simulink model "tp1"  (R2017b)
settings: Solver=VariableStepAuto  StartTime=0.0  StopTime=10.0  RelTol=1e-3
values from neighbouring files (symbols this model uses):
  A = [0 1 0;0 0 1;-2 -5 -4]    [TP1.m]
  a1 = 10    [TP1.m]
  a2 = 20    [TP1.m]
  a3 = 40    [TP1.m]
  B = [0;0;1]    [TP1.m]
  C = [1 0 0]    [TP1.m]
  F = exp(1)^A*T    [TP1.m]
  H = C    [TP1.m]
  L = [place(A',C',P)]'    [TP1.m]
  l1 = 25    [TP1.m]
  l2 = 20    [TP1.m]
  l3 = 35    [TP1.m]
undefined symbols (not defined in the file or in its folder): G
libraries: dspsrcs4 x2
settings Model: Creator=dell 15  LastModifiedBy=bo199

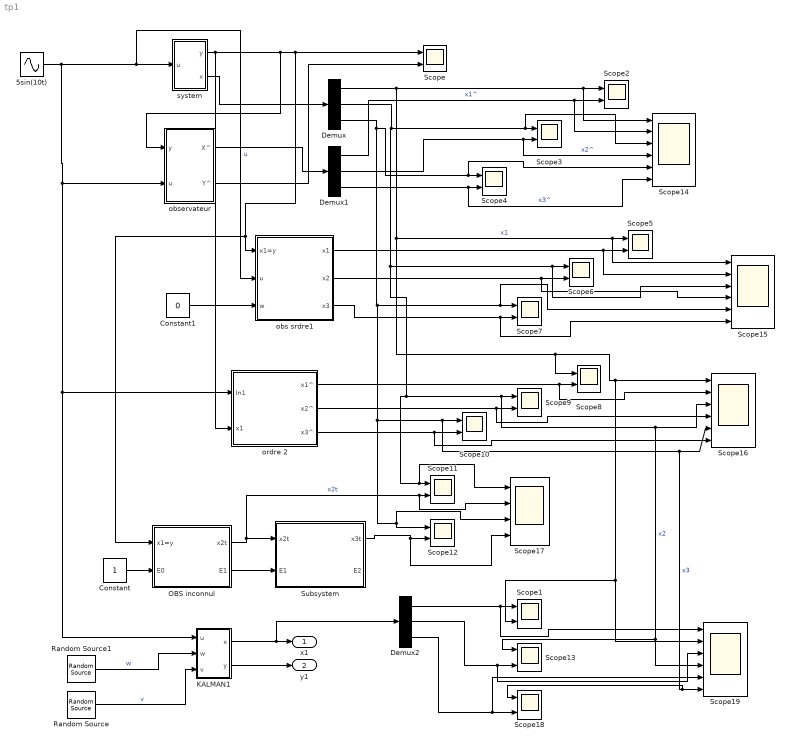
== system tp1 ==
  5sin(10t) : Sin  Amplitude=5  Frequency=10  SampleTime=0
  Constant : Constant
  Constant1 : Constant  Value=0
  Demux : Demux  Outputs=3
  Demux1 : Demux  Outputs=3
  Demux2 : Demux  Outputs=3
  KALMAN1 : Subsystem
  OBS inconnul : Subsystem
  Random Source : dspsrcs4/Random Source  SrcType=Uniform  NormMethod=Ziggurat  CltLength=12  MinVal=0  MaxVal=1  MeanVal=0  VarVal=1  RepMode=Not repeatable  rawSeed=1  IsInherit=off  SampMode=Discrete  SampTime=1  SampFrame=1  DataType=Double  OutComplex=Real  OutputFrames=off
  Random Source1 : dspsrcs4/Random Source  SrcType=Uniform  NormMethod=Ziggurat  CltLength=12  MinVal=0  MaxVal=1  MeanVal=0  VarVal=1  RepMode=Not repeatable  rawSeed=1  IsInherit=off  SampMode=Discrete  SampTime=1  SampFrame=1  DataType=Double  OutComplex=Real  OutputFrames=off
  Scope{,1..13,18} (15 alike) : Scope  NumInputPorts=2
  Scope{14..16,19} (4 alike) : Scope  NumInputPorts=6
  Scope17 : Scope  NumInputPorts=4
  Subsystem : Subsystem
  obs srdre1 : Subsystem
  observateur : Subsystem
  "ordre 2 " : Subsystem
  system : Subsystem
  x1 : Outport
  y1 : Outport  Port=2
  wires:
  system/1(y) -> Scope/1, OBS inconnul/1(x1=y), obs srdre1/1(x1=y), observateur/1(y), "ordre 2 "/2("x1 ")
  5sin(10t)/1 -> "ordre 2 "/1(In1), KALMAN1/1(u), observateur/2(u), obs srdre1/2(u), system/1("u ")  "u"
  system/2(x) -> Demux/1
  observateur/2(Y^) -> Scope/2
  OBS inconnul/1(x2t) -> Subsystem/1(x2t), Scope17/2, Scope11/2  "x2t"
  OBS inconnul/2(E1) -> Subsystem/2(E1)
  Constant/1 -> OBS inconnul/2(E0)
  Random Source1/1 -> KALMAN1/2(w)  "w"
  Random Source/1 -> KALMAN1/3(v)  "v"
  KALMAN1/2(y) -> y1/1
  Demux/3 -> Scope17/3, Scope12/1, Scope18/1, Scope19/6, Scope16/5, Scope10/1, Scope15/5, Scope7/1, Scope14/5, Scope4/1  "x3"
  Demux/2 -> Scope19/4, Scope13/1, Scope16/3, Scope9/1, Scope17/1, Scope11/1, Scope15/3, Scope6/1, Scope14/3, Scope3/1  "x2"
  Demux/1 -> Scope8/1, Scope19/2, Scope1/2, Scope16/1, Scope15/1, Scope5/1, Scope14/1, Scope2/1  "x1"
  observateur/1(X^) -> Demux1/1
  Demux1/1 -> Scope14/2, Scope2/2  "x1^"
  Demux1/2 -> Scope14/4, Scope3/2  "x2^"
  Demux1/3 -> Scope14/6, Scope4/2  "x3^"
  obs srdre1/1(x1) -> Scope15/2, Scope5/2
  obs srdre1/2(x2) -> Scope15/4, Scope6/2
  obs srdre1/3(x3) -> Scope15/6, Scope7/2
  "ordre 2 "/1(x1^) -> Scope16/2, Scope8/2
  "ordre 2 "/2(x2^) -> Scope16/4, Scope9/2
  "ordre 2 "/3(x3^) -> Scope16/6, Scope10/2
  Constant1/1 -> obs srdre1/3(w)
  Subsystem/1(x3t) -> Scope17/4, Scope12/2
  KALMAN1/1(x) -> Demux2/1, x1/1
  Demux2/1 -> Scope19/1, Scope1/1
  Demux2/2 -> Scope19/3, Scope13/2
  Demux2/3 -> Scope19/5, Scope18/2

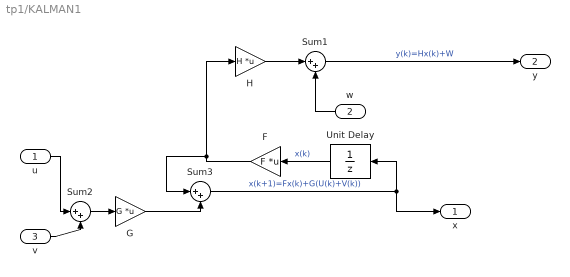
== system tp1/KALMAN1 ==
  u : Inport
  w : Inport  Port=2
  v : Inport  Port=3
  F : Gain  Gain=F  Multiplication=Matrix(K*u)
  G : Gain  Gain=G  Multiplication=Matrix(K*u)
  H : Gain  Gain=H  Multiplication=Matrix(K*u)
  Sum1 : Sum  Inputs=|++
  Sum2 : Sum  Inputs=|++
  Sum3 : Sum  Inputs=|++
  Unit Delay : UnitDelay  SampleTime=-1
  x : Outport
  y : Outport  Port=2
  wires:
  Sum3/1 -> x/1, Unit Delay/1  "x(k+1)=Fx(k)+G(U(k)+V(k))"
  F/1 -> H/1, Sum3/1
  u/1 -> Sum2/1
  Sum1/1 -> y/1  "y(k)=Hx(k)+W"
  H/1 -> Sum1/1
  G/1 -> Sum3/2
  Unit Delay/1 -> F/1  "x(k)"
  v/1 -> Sum2/2
  Sum2/1 -> G/1
  w/1 -> Sum1/2

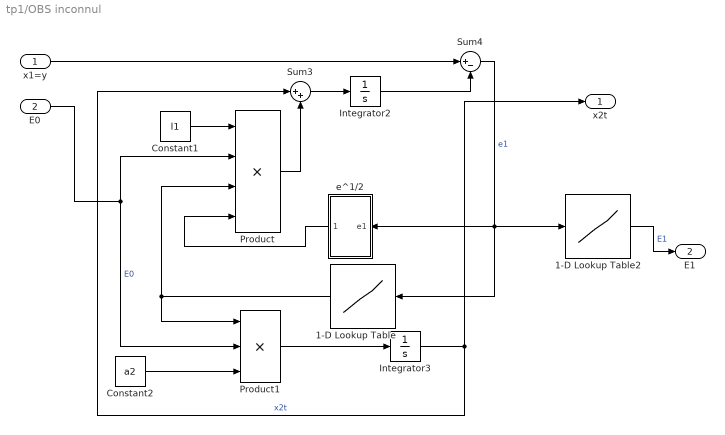
== system tp1/OBS inconnul ==
  x1=y : Inport
  E0 : Inport  Port=2
  1-D Lookup Table : Lookup_n-D  NumberOfTableDimensions=1  BreakpointsForDimension1=[-500 -0.011 -0.01 0.01 0.011 500]  Table=[-1 -1 -1 1 1 1 ]  InternalRulePriority=Speed  RndMeth=Simplest  InputSameDT=on
  1-D Lookup Table2 : Lookup_n-D  NumberOfTableDimensions=1  BreakpointsForDimension1=[-500 -0.011 -0.01 0.01 0.011 500]  Table=[0 0 1 1 0 0 ]  InternalRulePriority=Speed  RndMeth=Simplest  InputSameDT=on
  Constant1 : Constant  Value=l1
  Constant2 : Constant  Value=a2
  Integrator2 : Integrator
  Integrator3 : Integrator
  Product : Product  Inputs=4
  Product1 : Product  Inputs=3
  Sum3 : Sum  Inputs=|++
  Sum4 : Sum  Inputs=|+-
  e^1/2 : Subsystem
  x2t : Outport
  E1 : Outport  Port=2
  wires:
  1-D Lookup Table2/1 -> E1/1  "E1"
  e^1/2/1(Out1) -> Product/4
  x1=y/1 -> Sum4/1
  Integrator3/1 -> x2t/1, Sum3/1  "x2t"
  Sum3/1 -> Integrator2/1
  Product/1 -> Sum3/2
  Product1/1 -> Integrator3/1
  E0/1 -> Product1/2, Product/2  "E0"
  Integrator2/1 -> Sum4/2
  Constant1/1 -> Product/1
  Constant2/1 -> Product1/3
  Sum4/1 -> 1-D Lookup Table/1, e^1/2/1(e1), 1-D Lookup Table2/1  "e1"
  1-D Lookup Table/1 -> Product/3, Product1/1

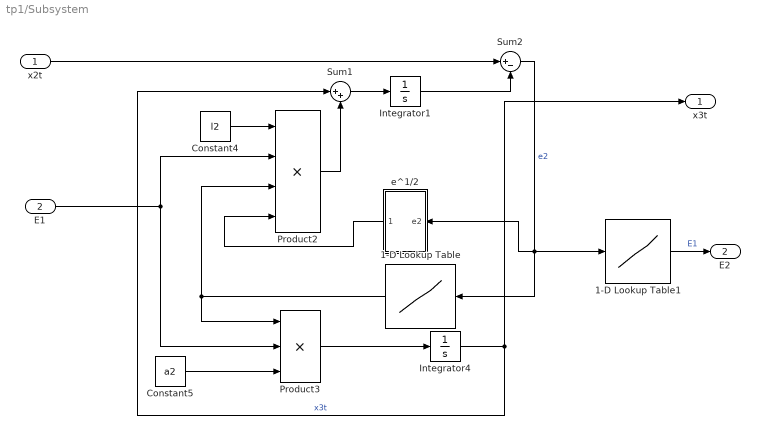
== system tp1/Subsystem ==
  x2t : Inport
  E1 : Inport  Port=2
  1-D Lookup Table : Lookup_n-D  NumberOfTableDimensions=1  BreakpointsForDimension1=[-500 -0.011 -0.01 0.01 0.011 500]  Table=[-1 -1 -1 1 1 1 ]  InternalRulePriority=Speed  RndMeth=Simplest  InputSameDT=on
  1-D Lookup Table1 : Lookup_n-D  NumberOfTableDimensions=1  BreakpointsForDimension1=[-500 -0.011 -0.01 0.01 0.011 500]  Table=[0 0 1 1 0 0 ]  InternalRulePriority=Speed  RndMeth=Simplest  InputSameDT=on
  Constant4 : Constant  Value=l2
  Constant5 : Constant  Value=a2
  Integrator1 : Integrator
  Integrator4 : Integrator
  Product2 : Product  Inputs=4
  Product3 : Product  Inputs=3
  Sum1 : Sum  Inputs=|++
  Sum2 : Sum  Inputs=|+-
  e^1/2 : Subsystem
  x3t : Outport
  E2 : Outport  Port=2
  wires:
  e^1/2/1(Out1) -> Product2/4
  x2t/1 -> Sum2/1
  Integrator4/1 -> x3t/1, Sum1/1  "x3t"
  Integrator1/1 -> Sum2/2
  1-D Lookup Table/1 -> Product2/3, Product3/1
  Sum2/1 -> 1-D Lookup Table/1, e^1/2/1(e2), 1-D Lookup Table1/1  "e2"
  Product2/1 -> Sum1/2
  Product3/1 -> Integrator4/1
  1-D Lookup Table1/1 -> E2/1  "E1"
  Sum1/1 -> Integrator1/1
  E1/1 -> Product2/2, Product3/2
  Constant5/1 -> Product3/3
  Constant4/1 -> Product2/1

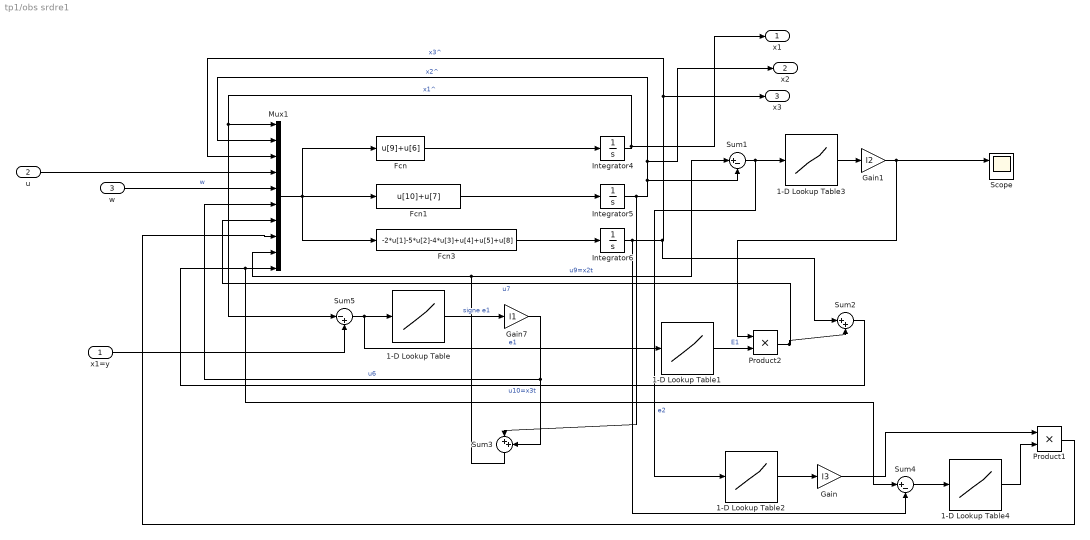
== system tp1/obs srdre1 ==
  x1=y : Inport
  u : Inport  Port=2
  w : Inport  Port=3
  1-D Lookup Table : Lookup_n-D  NumberOfTableDimensions=1  BreakpointsForDimension1=[-500 -0.011 -0.01 0.01 0.011 500]  Table=[-1 -1 -1 1 1 1 ]  InternalRulePriority=Speed  RndMeth=Simplest  InputSameDT=on
  1-D Lookup Table1 : Lookup_n-D  NumberOfTableDimensions=1  BreakpointsForDimension1=[-500 -0.011 -0.01 0.01 0.011 500]  Table=[0 0 1 1 0 0 ]  InternalRulePriority=Speed  RndMeth=Simplest  InputSameDT=on
  1-D Lookup Table2 : Lookup_n-D  NumberOfTableDimensions=1  BreakpointsForDimension1=[-500 -0.011 -0.01 0.01 0.011 500]  Table=[0 0 1 1 0 0 ]  InternalRulePriority=Speed  RndMeth=Simplest  InputSameDT=on
  1-D Lookup Table3 : Lookup_n-D  NumberOfTableDimensions=1  BreakpointsForDimension1=[-500 -0.011 -0.01 0.01 0.011 500]  Table=[-1 -1 -1 1 1 1 ]  InternalRulePriority=Speed  RndMeth=Simplest  InputSameDT=on
  1-D Lookup Table4 : Lookup_n-D  NumberOfTableDimensions=1  BreakpointsForDimension1=[-500 -0.011 -0.01 0.01 0.011 500]  Table=[-1 -1 -1 1 1 1 ]  InternalRulePriority=Speed  RndMeth=Simplest  InputSameDT=on
  Fcn : Fcn  Expr=u[9]+u[6]
  Fcn1 : Fcn  Expr=u[10]+u[7]
  Fcn3 : Fcn  Expr=-2*u[1]-5*u[2]-4*u[3]+u[4]+u[5]+u[8]
  Gain : Gain  Gain=l3
  Gain1 : Gain  Gain=l2
  Gain7 : Gain  Gain=l1
  Integrator4 : Integrator
  Integrator5 : Integrator
  Integrator6 : Integrator
  Mux1 : Mux  Inputs=10
  Product1 : Product
  Product2 : Product
  Scope : Scope  NumInputPorts=2
  Sum1 : Sum  Inputs=|+-
  Sum2 : Sum  Inputs=|++
  Sum3 : Sum  Inputs=|++
  Sum4 : Sum  Inputs=|+-
  Sum5 : Sum  Inputs=|-+
  x1 : Outport
  x2 : Outport  Port=2
  x3 : Outport  Port=3
  wires:
  Sum3/1 -> Mux1/9, Sum1/1  "u9=x2t"
  x1=y/1 -> Sum5/2
  u/1 -> Mux1/4
  Integrator6/1 -> Sum4/2, Sum2/1, x3/1, Mux1/3  "x3^"
  Mux1/1 -> Fcn/1, Fcn1/1, Fcn3/1
  1-D Lookup Table1/1 -> Product2/2  "E1"
  Fcn1/1 -> Integrator5/1
  Fcn3/1 -> Integrator6/1
  Integrator5/1 -> Sum1/2, x2/1, Mux1/2, Sum3/1  "x2^"
  Gain7/1 -> Mux1/6, Sum3/2  "u6"
  1-D Lookup Table/1 -> Gain7/1  "signe e1"
  Sum2/1 -> Sum4/1, Mux1/10  "u10=x3t"
  Product2/1 -> Sum2/2, Mux1/7  "u7"
  w/1 -> Mux1/5  "w"
  Fcn/1 -> Integrator4/1
  Integrator4/1 -> x1/1, Sum5/1, Mux1/1  "x1^"
  Sum5/1 -> 1-D Lookup Table1/1, 1-D Lookup Table/1  "e1"
  Gain1/1 -> Product2/1, Scope/1
  Sum1/1 -> 1-D Lookup Table2/1, 1-D Lookup Table3/1  "e2"
  1-D Lookup Table3/1 -> Gain1/1
  1-D Lookup Table2/1 -> Gain/1
  Sum4/1 -> 1-D Lookup Table4/1
  1-D Lookup Table4/1 -> Product1/2
  Gain/1 -> Product1/1
  Product1/1 -> Mux1/8

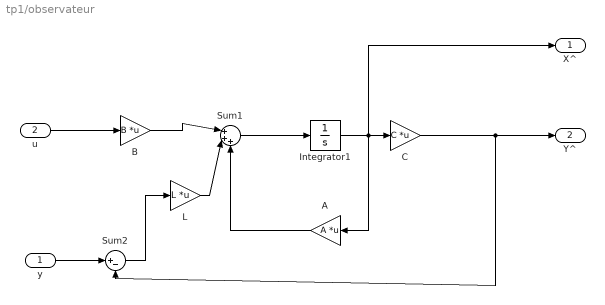
== system tp1/observateur ==
  y : Inport
  u : Inport  Port=2
  A : Gain  Gain=A  Multiplication=Matrix(K*u) (u vector)
  B : Gain  Gain=B  Multiplication=Matrix(K*u) (u vector)
  C : Gain  Gain=C  Multiplication=Matrix(K*u) (u vector)
  Integrator1 : Integrator  InitialCondition=[2 4 6]
  L : Gain  Gain=L  Multiplication=Matrix(K*u) (u vector)
  Sum1 : Sum  Inputs=|+++
  Sum2 : Sum  Inputs=|+-
  X^ : Outport
  Y^ : Outport  Port=2
  wires:
  u/1 -> B/1
  y/1 -> Sum2/1
  C/1 -> Y^/1, Sum2/2
  Sum2/1 -> L/1
  A/1 -> Sum1/3
  Sum1/1 -> Integrator1/1
  B/1 -> Sum1/1
  Integrator1/1 -> X^/1, A/1, C/1
  L/1 -> Sum1/2

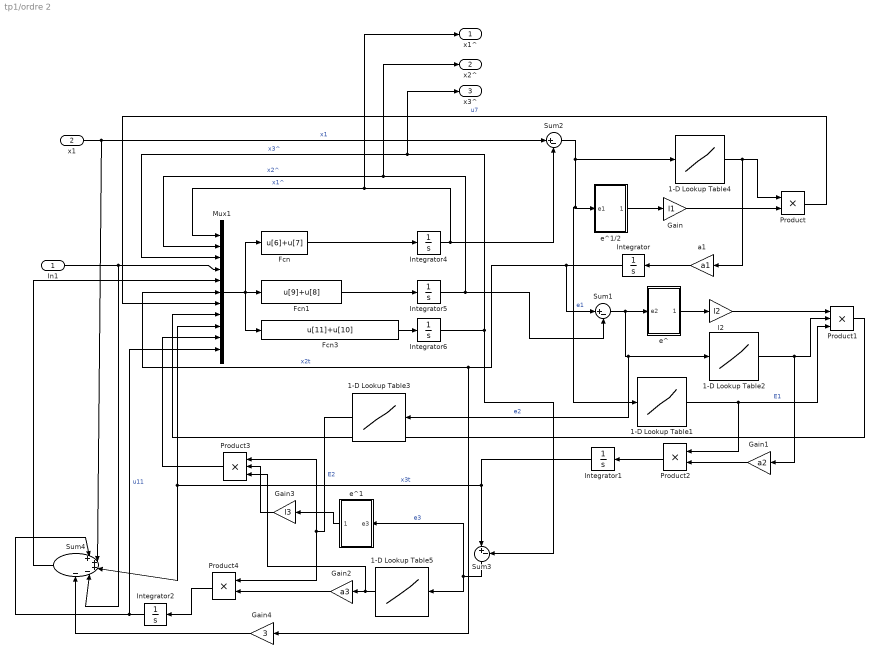
== system tp1/ordre 2  ==
  In1 : Inport
  "x1 " : Inport  Port=2
  1-D Lookup Table1 : Lookup_n-D  NumberOfTableDimensions=1  BreakpointsForDimension1=[-500 -0.011 -0.01 0.01 0.011 500]  Table=[0 0 1 1 0 0 ]  InternalRulePriority=Speed  RndMeth=Simplest  InputSameDT=on
  1-D Lookup Table2 : Lookup_n-D  NumberOfTableDimensions=1  BreakpointsForDimension1=[-500 -0.011 -0.01 0.01 0.011 500]  Table=[-1 -1 -1 1 1 1 ]  InternalRulePriority=Speed  RndMeth=Simplest  InputSameDT=on
  1-D Lookup Table3 : Lookup_n-D  NumberOfTableDimensions=1  BreakpointsForDimension1=[-500 -0.011 -0.01 0.01 0.011 500]  Table=[0 0 1 1 0 0 ]  InternalRulePriority=Speed  RndMeth=Simplest  InputSameDT=on
  1-D Lookup Table4 : Lookup_n-D  NumberOfTableDimensions=1  BreakpointsForDimension1=[-500 -0.011 -0.01 0.01 0.011 500]  Table=[-1 -1 -1 1 1 1 ]  InternalRulePriority=Speed  RndMeth=Simplest  InputSameDT=on
  1-D Lookup Table5 : Lookup_n-D  NumberOfTableDimensions=1  BreakpointsForDimension1=[-500 -0.011 -0.01 0.01 0.011 500]  Table=[-1 -1 -1 1 1 1 ]  InternalRulePriority=Speed  RndMeth=Simplest  InputSameDT=on
  Fcn : Fcn  Expr=u[6]+u[7]
  Fcn1 : Fcn  Expr=u[9]+u[8]
  Fcn3 : Fcn  Expr=u[11]+u[10]
  Gain : Gain  Gain=l1
  Gain1 : Gain  Gain=a2
  Gain2 : Gain  Gain=a3
  Gain3 : Gain  Gain=l3
  Gain4 : Gain  Gain=3
  Integrator{,1..2,4..6} (6 alike) : Integrator
  Mux1 : Mux  Inputs=11
  Product : Product
  Product1 : Product  Inputs=3
  Product2 : Product
  Product3 : Product  Inputs=3
  Product4 : Product
  Sum1 : Sum  Inputs=|+-
  Sum2 : Sum  Inputs=|+-
  Sum3 : Sum  Inputs=|+-
  Sum4 : Sum  Inputs=|+++--
  a1 : Gain  Gain=a1
  e^ : Subsystem
  e^1 : Subsystem
  e^1/2 : Subsystem
  l2 : Gain  Gain=l2
  x1^ : Outport
  x2^ : Outport  Port=2
  x3^ : Outport  Port=3
  wires:
  Fcn1/1 -> Integrator5/1
  Sum4/1 -> Mux1/5
  Integrator5/1 -> x2^/1, Mux1/2, Sum1/2  "x2^"
  Mux1/1 -> Fcn/1, Fcn1/1, Fcn3/1
  Integrator6/1 -> Sum3/2, x3^/1, Mux1/3  "x3^"
  Fcn/1 -> Integrator4/1
  Integrator4/1 -> Sum2/2, x1^/1, Mux1/1  "x1^"
  Fcn3/1 -> Integrator6/1
  Product3/1 -> Mux1/10
  Product/1 -> Mux1/7  "u7"
  Integrator1/1 -> Sum4/3, Mux1/9, Sum3/1  "x3t"
  Product1/1 -> Mux1/8
  Integrator/1 -> Sum1/1, Gain4/1, Mux1/6  "x2t"
  e^1/2/1(Out1) -> Gain/1
  Sum2/1 -> 1-D Lookup Table1/1, e^1/2/1(e1), 1-D Lookup Table4/1  "e1"
  "x1 "/1 -> Sum2/1, Sum4/2  "x1"
  Gain/1 -> Product/2
  1-D Lookup Table4/1 -> a1/1, Product/1
  a1/1 -> Integrator/1
  Sum1/1 -> 1-D Lookup Table3/1, 1-D Lookup Table2/1, e^/1(e2)  "e2"
  e^/1(Out1) -> l2/1
  1-D Lookup Table2/1 -> Gain1/1, Product1/2
  l2/1 -> Product1/1
  1-D Lookup Table1/1 -> Product1/3, Product2/1  "E1"
  Gain1/1 -> Product2/2
  Product2/1 -> Integrator1/1
  1-D Lookup Table3/1 -> Product4/1, Product3/1  "E2"
  Sum3/1 -> 1-D Lookup Table5/1, e^1/1(e3)  "e3"
  Gain2/1 -> Product4/2
  1-D Lookup Table5/1 -> Product3/3, Gain2/1
  Product4/1 -> Integrator2/1
  Integrator2/1 -> Mux1/11, Sum4/1  "u11"
  e^1/1(Out1) -> Gain3/1
  Gain3/1 -> Product3/2
  Gain4/1 -> Sum4/5
  In1/1 -> Sum4/4, Mux1/4

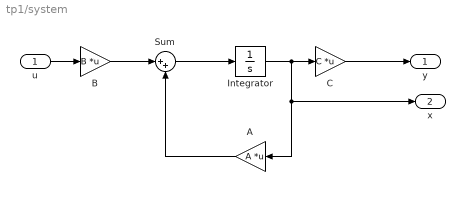
== system tp1/system ==
  "u " : Inport
  A : Gain  Gain=A  Multiplication=Matrix(K*u) (u vector)
  B : Gain  Gain=B  Multiplication=Matrix(K*u) (u vector)
  C : Gain  Gain=C  Multiplication=Matrix(K*u) (u vector)
  Integrator : Integrator  InitialCondition=[1 2 3]
  Sum : Sum  Inputs=|++
  y : Outport
  x : Outport  Port=2
  wires:
  "u "/1 -> B/1
  Integrator/1 -> x/1, A/1, C/1
  A/1 -> Sum/2
  B/1 -> Sum/1
  Sum/1 -> Integrator/1
  C/1 -> y/1

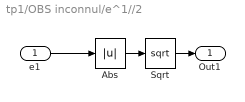
== system tp1/OBS inconnul/e^1//2 ==
  e1 : Inport
  Abs : Abs
  Sqrt : Sqrt  SaturateOnIntegerOverflow=on
  Out1 : Outport
  wires:
  Sqrt/1 -> Out1/1
  e1/1 -> Abs/1
  Abs/1 -> Sqrt/1

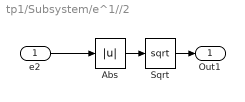
== system tp1/Subsystem/e^1//2 ==
  e2 : Inport
  Abs : Abs
  Sqrt : Sqrt  SaturateOnIntegerOverflow=on
  Out1 : Outport
  wires:
  Sqrt/1 -> Out1/1
  e2/1 -> Abs/1
  Abs/1 -> Sqrt/1

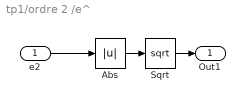
== system tp1/ordre 2 /e^ ==
  e2 : Inport
  Abs : Abs
  Sqrt : Sqrt  SaturateOnIntegerOverflow=on
  Out1 : Outport
  wires:
  Sqrt/1 -> Out1/1
  e2/1 -> Abs/1
  Abs/1 -> Sqrt/1

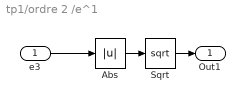
== system tp1/ordre 2 /e^1 ==
  e3 : Inport
  Abs : Abs
  Sqrt : Sqrt  SaturateOnIntegerOverflow=on
  Out1 : Outport
  wires:
  Sqrt/1 -> Out1/1
  e3/1 -> Abs/1
  Abs/1 -> Sqrt/1

== system tp1/ordre 2 /e^1//2 ==
  e1 : Inport
  Abs : Abs
  Sqrt : Sqrt  SaturateOnIntegerOverflow=on
  Out1 : Outport
  wires:
  Sqrt/1 -> Out1/1
  e1/1 -> Abs/1
  Abs/1 -> Sqrt/1
